simulink model "Resolver_PLL_2022a_JAS"  (R2022b)
settings: Solver=FixedStepAuto  StartTime=0.0  StopTime=0.04  FixedStep=1e-7  RelTol=1e-3
InitFcn:
  | Pole_pairs =2
  | alphaOne= 0.59724
  | alphaTwo = 0.92835
  | alphaThree = 0.25059
  | Wo = 5000
  | qOne = alphaOne*Wo
  | qTwo = alphaTwo*Wo*Wo
  | qThree = alphaThree*Wo*Wo*Wo
  | dampening = 3
undefined symbols (not defined in the file): DiscIntNeverNeededParam
libraries: dspsigops x2, simulink x1, dsparch4 x1
settings Model: Creator=e36916  LastModifiedBy=randa

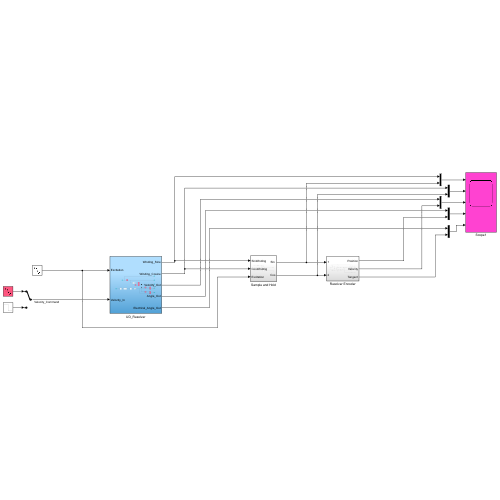
[thumbnail: Simulink's stored preview of the top-level diagram]
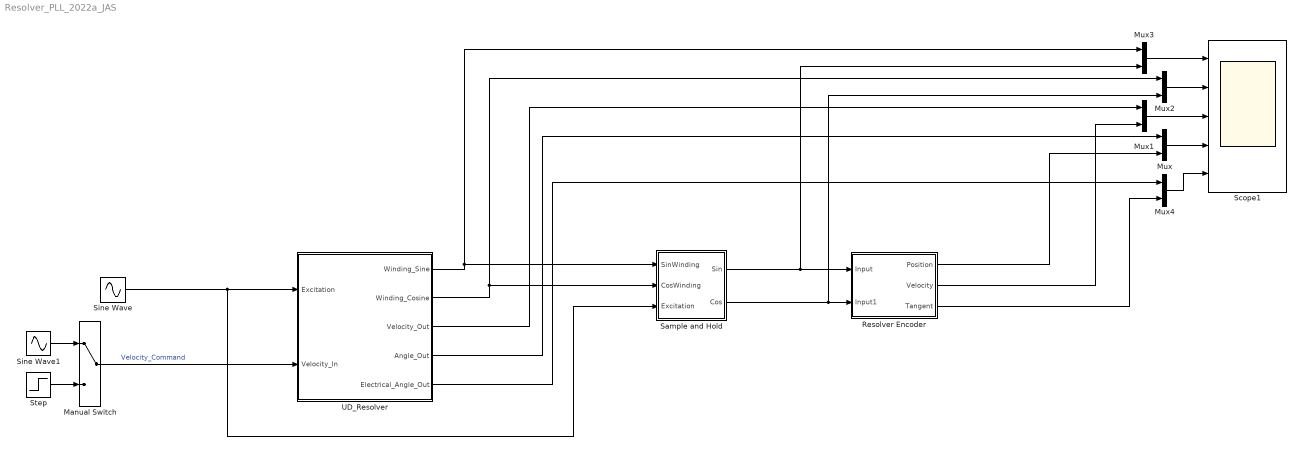
== system Resolver_PLL_2022a_JAS ==
  Manual Switch : ManualSwitch
  Mux{,1..4} (5 alike) : Mux  Inputs=2
  Resolver Encoder : Subsystem
  Sample and Hold : Subsystem
  Scope1 : Scope  NumInputPorts=5
  Sine Wave : Sin  Amplitude=1.36  Bias=1.36  Frequency=2*pi*10000
  Sine Wave1 : Sin  Amplitude=3000  Frequency=50*pi  SampleTime=0
  Step : Step  Time=0.02  Before=100  After=0  SampleTime=0
  UD_Resolver : Subsystem
  wires:
  UD_Resolver/1(Winding_Sine) -> Mux3/1, Sample and Hold/1(SinWinding)
  Sine Wave/1 -> Sample and Hold/3(Excitation), UD_Resolver/1(Excitation)
  Sine Wave1/1 -> Manual Switch/1
  Manual Switch/1 -> UD_Resolver/2(Velocity_In)  "Velocity_Command"
  Step/1 -> Manual Switch/2
  UD_Resolver/2(Winding_Cosine) -> Sample and Hold/2(CosWinding), Mux2/1
  Mux/1 -> Scope1/4
  UD_Resolver/4(Angle_Out) -> Mux/1
  Resolver Encoder/1(Position) -> Mux/2
  Mux1/1 -> Scope1/3
  UD_Resolver/3(Velocity_Out) -> Mux1/1
  Mux2/1 -> Scope1/2
  Mux3/1 -> Scope1/1
  Sample and Hold/2(" Cos") -> Resolver Encoder/2(Input1), Mux2/2
  Sample and Hold/1("Sin ") -> Resolver Encoder/1(Input), Mux3/2
  Mux4/1 -> Scope1/5
  Resolver Encoder/3(Tangent) -> Mux4/2
  UD_Resolver/5(Electrical_Angle_Out) -> Mux4/1
  Resolver Encoder/2(Velocity) -> Mux1/2

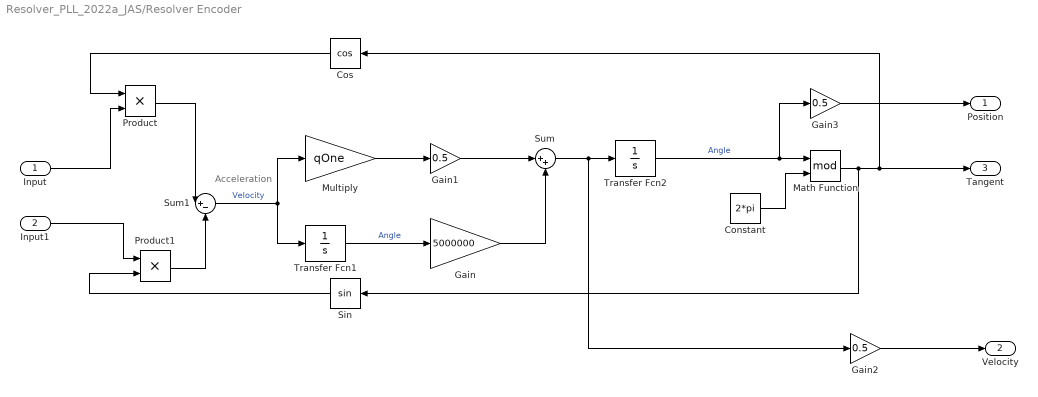
== system Resolver_PLL_2022a_JAS/Resolver Encoder ==
  note: Acceleration
  Input : Inport
  Input1 : Inport  Port=2
  Constant : Constant  Value=2*pi
  Cos : Trigonometry  Operator=cos
  Gain : Gain  Gain=5000000
  Gain1 : Gain  Gain=0.5
  Gain2 : Gain  Gain=0.5
  Gain3 : Gain  Gain=0.5
  Math Function : Math  Operator=mod
  Multiply : Gain  Gain=qOne
  Product : Product
  Product1 : Product
  Sin : Trigonometry
  Sum : Sum  Inputs=|++
  Sum1 : Sum  Inputs=|+-
  Transfer Fcn1 : TransferFcn  Denominator=[1 0]
  Transfer Fcn2 : TransferFcn  Denominator=[1 0]
  Position : Outport
  Velocity : Outport  Port=2
  Tangent : Outport  Port=3
  wires:
  Sum1/1 -> Transfer Fcn1/1, Multiply/1  "Velocity"
  Product/1 -> Sum1/1
  Transfer Fcn2/1 -> Gain3/1, Math Function/1  "Angle"
  Sum/1 -> Gain2/1, Transfer Fcn2/1
  Sin/1 -> Product1/2
  Product1/1 -> Sum1/2
  Multiply/1 -> Gain1/1
  Cos/1 -> Product/1
  Input/1 -> Product/2
  Input1/1 -> Product1/1
  Gain/1 -> Sum/2
  Gain1/1 -> Sum/1
  Math Function/1 -> Sin/1, Tangent/1, Cos/1
  Constant/1 -> Math Function/2
  Gain2/1 -> Velocity/1
  Transfer Fcn1/1 -> Gain/1  "Angle"
  Gain3/1 -> Position/1

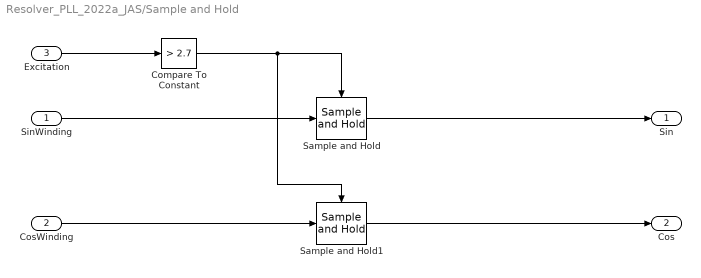
== system Resolver_PLL_2022a_JAS/Sample and Hold ==
  SinWinding : Inport
  CosWinding : Inport  Port=2
  Excitation : Inport  Port=3
  Compare To Constant : simulink/Logic and Bit Operations/Compare To Constant  relop=>  const=2.7  OutDataTypeStr=boolean
  Sample and Hold : dspsigops/Sample and Hold  trig=Rising edge  initCond=0  latchinput=off
  Sample and Hold1 : dspsigops/Sample and Hold  trig=Rising edge  initCond=0  latchinput=off
  "Sin " : Outport
  " Cos" : Outport  Port=2
  wires:
  CosWinding/1 -> Sample and Hold1/1
  SinWinding/1 -> Sample and Hold/1
  Excitation/1 -> Compare To Constant/1
  Compare To Constant/1 -> Sample and Hold1/Trigger, Sample and Hold/Trigger
  Sample and Hold/1 -> "Sin "/1
  Sample and Hold1/1 -> " Cos"/1

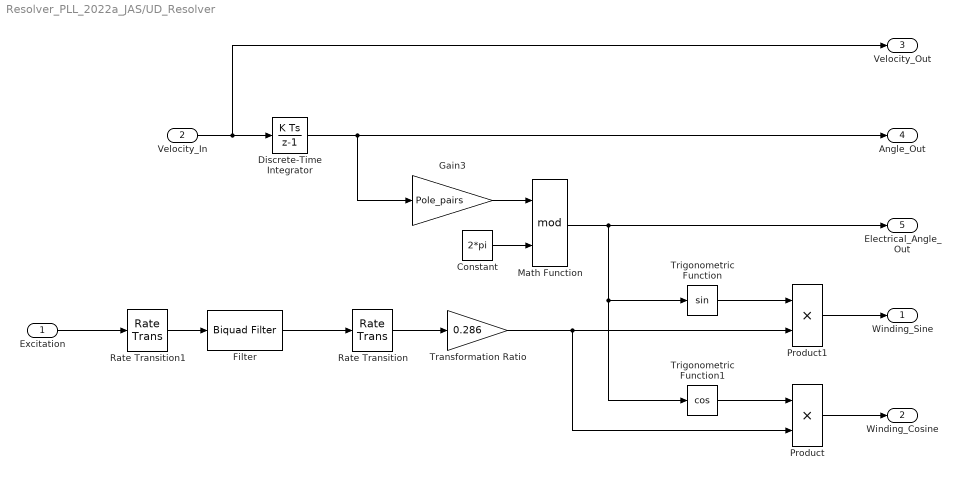
== system Resolver_PLL_2022a_JAS/UD_Resolver ==
  Excitation : Inport
  Velocity_In : Inport  Port=2
  Constant : Constant  Value=2*pi
  Discrete-Time Integrator : DiscreteIntegrator  SampleTime=-1  ICPrevOutput=DiscIntNeverNeededParam  ICPrevScaledInput=DiscIntNeverNeededParam
  Filter : dsparch4/Biquad Filter  Tag=BlockMethodSubSystem  FilterSource=Dialog parameters  CoeffSource=Specify via dialog  FilterObject=BQF  IIRFiltStruct=Direct form II  BiQuadCoeffs=[1 -2 1 1 -1.98532458709362158 0.98567733794518908;1 -2 1 1 -1.96541950338359084 0.965768717516137798]  ScaleValues=[0.992750481259702666;0.982797055224932214;1]  IC=0  ICnum=0  ICden=0  a0Flag=Warning  optimizeScaleValues=on  ScaleValueMode=Specify via input port (g)  InputProcessing=Columns as channels (frame based)  roundingMode=Floor  overflowMode=off  scaleValueFracLength=14  denProdOutputFracLength=30  denAccumFracLength=30  secondMemoryFracLength=15
  Gain3 : Gain  Gain=Pole_pairs
  Math Function : Math  Operator=mod
  Product : Product
  Product1 : Product
  Rate Transition : RateTransition  OutPortSampleTime=1e-7
  Rate Transition1 : RateTransition  OutPortSampleTime=1/1000000
  Transformation Ratio : Gain  Gain=0.286
  Trigonometric Function : Trigonometry
  Trigonometric Function1 : Trigonometry  Operator=cos
  Winding_Sine : Outport  VectorParamsAs1DForOutWhenUnconnected=off
  Winding_Cosine : Outport  Port=2  VectorParamsAs1DForOutWhenUnconnected=off
  Velocity_Out : Outport  Port=3  VectorParamsAs1DForOutWhenUnconnected=off
  Angle_Out : Outport  Port=4  VectorParamsAs1DForOutWhenUnconnected=off
  Electrical_Angle_Out : Outport  Port=5  VectorParamsAs1DForOutWhenUnconnected=off
  wires:
  Velocity_In/1 -> Velocity_Out/1, Discrete-Time Integrator/1
  Product1/1 -> Winding_Sine/1
  Transformation Ratio/1 -> Product/2, Product1/2
  Product/1 -> Winding_Cosine/1
  Excitation/1 -> Rate Transition1/1
  Discrete-Time Integrator/1 -> Angle_Out/1, Gain3/1
  Constant/1 -> Math Function/2
  Math Function/1 -> Electrical_Angle_Out/1, Trigonometric Function/1, Trigonometric Function1/1
  Gain3/1 -> Math Function/1
  Trigonometric Function/1 -> Product1/1
  Trigonometric Function1/1 -> Product/1
  Rate Transition1/1 -> Filter/1
  Rate Transition/1 -> Transformation Ratio/1
  Filter/1 -> Rate Transition/1
